simulink model "Maglev_SMC_mfunc"  (R2025a)
settings: Solver=ode23t  StartTime=0.0  StopTime=T_sim  FixedStep=ekf_params.Ts  MaxStep=Ts  RelTol=1e-2  AbsTol=1e-4
PreLoadFcn:
  | % Modellpfad abrufen
  | modelPath = fileparts(which(bdroot));
  | projectRoot = fileparts(modelPath);
  | 
  | % Simulationsumgebung einrichten und Parameter laden
  | run(fullfile(projectRoot, 'setup_sim_params.m'));
  | load(fullfile(projectRoot, 'Controller_Params', 'EKFData.mat'));
  | load(fullfile(projectRoot, 'Controller_Params', 'NonlinearControllerData.mat'));
undefined symbols (not defined in the file): ekf_params, Ext_Fina_Val, Ext_Init_Val, grav, I_max, I_min, Km, mass, Plant, smc, T_stp
libraries: fl_lib x11, nesl_utility x4
settings Model: Creator=Polarstern  LastModifiedBy=CelestialAurora
settings DebuggingCC: AlgebraicLoopMsg=none

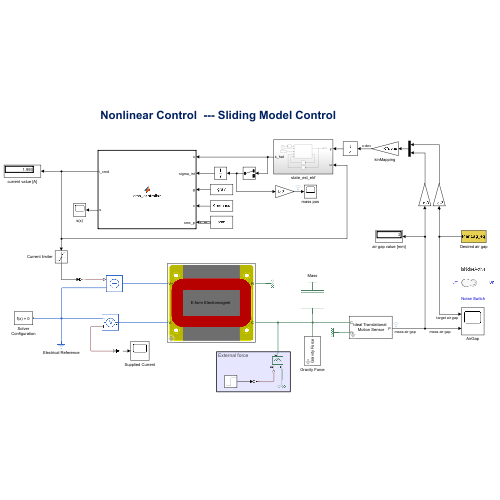
[thumbnail: Simulink's stored preview of the top-level diagram]
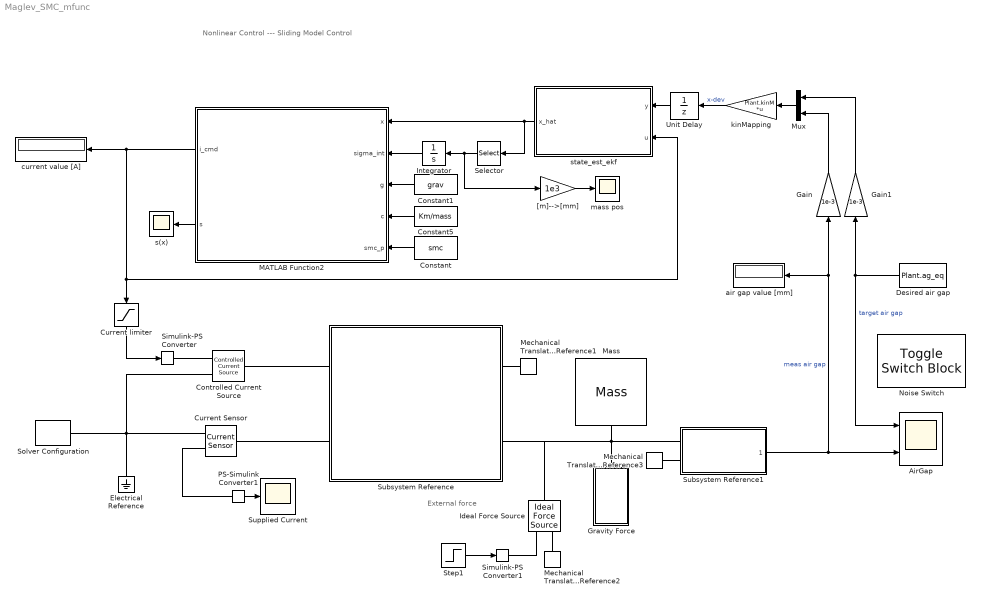
== system Maglev_SMC_mfunc ==
  note: External force
  note: Nonlinear Control --- Sliding Model Control
  AirGap : Scope  NumInputPorts=2
      settings: ActiveDisplayYMinimum=1.7979494790618245  ActiveDisplayYMaximum=2.5780056134375751
  Constant : Constant  Value=smc  OutDataTypeStr=Bus: smc_Bus
  Constant1 : Constant  Value=grav
  Constant5 : Constant  Value=Km/mass
  Controlled Current Source : fl_lib/Electrical/Electrical Sources/Controlled Current Source
  Current Sensor : fl_lib/Electrical/Electrical Sensors/Current Sensor
  Current limiter : Saturate  UpperLimit=I_max  LowerLimit=I_min
  Desired air gap : Constant  Value=Plant.ag_eq
  Electrical Reference : fl_lib/Electrical/Electrical Elements/Electrical Reference
  Gain : Gain  Gain=1e-3
  Gain1 : Gain  Gain=1e-3
  Gravity Force : Subsystem
      mask DialogControl DescGroupVar Prompt: Gravity Force
      mask DialogControl DescTextVar Prompt: Fg = Mass*grav, as constant parameters predefined
      mask DialogControl DescTextVar2 Prompt: Direction: Downward
      mask Display: disp("Gravity Force")
  Ideal Force Source : fl_lib/Mechanical/Mechanical Sources/Ideal Force Source
  Integrator : Integrator
  MATLAB Function2 : MATLAB Function  TreatAsAtomicUnit=on
  Mass : fl_lib/Mechanical/Translational Elements/Mass  mass=mass kg  num_ports=foundation.enum.numPorts2.one  v_specify=on  v_priority=Low  v=0 m/s  v_nominal_specify=off  v_nominal_value=1  v_nominal_unit=m/s  f_specify=off  f_priority=None  f=0 N  f_nominal_specify=off  f_nominal_value=700  f_nominal_unit=N
  Mechanical Translational Reference1 : fl_lib/Mechanical/Translational Elements/Mechanical Translational Reference
  Mechanical Translational Reference2 : fl_lib/Mechanical/Translational Elements/Mechanical Translational Reference
  Mechanical Translational Reference3 : fl_lib/Mechanical/Translational Elements/Mechanical Translational Reference
  Mux : Mux  Inputs=2
  Noise Switch : ToggleSwitchBlock
  PS-Simulink Converter1 : nesl_utility/PS-Simulink Converter  PhysicalDomain=network_engine_domain  SubClassName=ps_output  LeftPortType=input  RightPortType=output  PseudoPeriodic=off  Frequencies=[]  VectorFormat=inherit  Unit=inherit  AffineConversion=off
  Selector : Selector  InputPortWidth=2  IndexOptions=Index vector (dialog)  Indices=[1]  OutputSizes=1
  Simulink-PS Converter : nesl_utility/Simulink-PS Converter  PhysicalDomain=network_engine_domain  SubClassName=ps_input  LeftPortType=input  RightPortType=output  PseudoPeriodic=off  Frequencies=[]  NoiseDistribution=none  NoiseParameters=[]  Unit=1  AffineConversion=off  FilteringAndDerivatives=zero  SimscapeFilterOrder=1  InputFilterTimeConstant=0.001  UdotUserProvided=0
  Simulink-PS Converter1 : nesl_utility/Simulink-PS Converter  PhysicalDomain=network_engine_domain  SubClassName=ps_input  LeftPortType=input  RightPortType=output  PseudoPeriodic=off  Frequencies=[]  NoiseDistribution=none  NoiseParameters=[]  Unit=1  AffineConversion=off  FilteringAndDerivatives=provide  SimscapeFilterOrder=1  InputFilterTimeConstant=0.001  UdotUserProvided=0
  Solver Configuration : nesl_utility/Solver Configuration  PhysicalDomain=network_engine_domain  SubClassName=solver  LeftPortType=input  RightPortType=generic  Tones=[]  Harmonics=[]  SimulateNoise=off  Profile=off  UseLocalSampling=off  EnableSwitchedLinearOptims=on  FrequencyDomain=off  UseCCode=off  RelTol=0.001  AbsTol=1e-06  MinStep=1e-09  ToWorkspace=off  RevertToSquareIcSolve=off  NumHomotopyIterations=100  PhasorMode=off  PhasorModeNumHarmonics=1  ConsistencySolver=NEWTON_XTOL_AFTER_FTOL  IndexReductionMethod=DerivativeReplacement  DoDC=off  ResidualTolerance=1e-09  ConsistencyTolSource=GLOBAL  ConsistencyAbsTol=0.001  ConsistencyRelTol=0.001  ConsistencyTolFactor=0.001  UseLocalSolver=on  LocalSolverChoice=NE_BACKWARD_EULER_ADVANCER  ResolveIndetEquations=on  FunctionEvalNumThread=1  LocalSolverSampleTime=ekf_params.Ts  DoFixedCost=off  MaxNonlinIter=3  MaxModeIter=2  ComputeImpulses=off  ImpulseIterations=2  LinearAlgebra=auto  LinearAlgebraNumThread=0  EquationFormulation=NE_TIME_EF  DelaysMemoryBudget=1024  AutomaticFiltering=on  FilteringTimeConstant=0.001  PartitionStorageMethod=AS_NEEDED  PartitionMemoryBudget=1024  PartitionMethod=ROBUST  MultibodyUseLocalSolver=off  MultibodyLocalSolverChoice=ODE1  MultibodyLocalSolverSampleTime=0.001
  Step1 : Step  Time=T_stp  Before=Ext_Init_Val  After=Ext_Fina_Val  SampleTime=0
  Subsystem Reference : Subsystem  ReferencedSubsystem=IntegratedElectromagnet  l_airgap=airgap_init
  Subsystem Reference1 : Subsystem  ReferencedSubsystem=IdealTrans_MotionSensor  ns_sw=isNoiseActive  ns_pw=NoisePower  ts=Ts  init_pos=airgap_init
  Supplied Current : Scope
      settings: ActiveDisplayYMinimum=-1.1586536453243705  ActiveDisplayYMaximum=10.427882807919337  DataLoggingVariableName=ScopeData3
  Unit Delay : UnitDelay  SampleTime=-1  HasFrameUpgradeWarning=on
  "[m]-->[mm]" : Gain  Gain=1e3
  air gap value [mm] : Display
      settings: Decimation=4
  current value [A] : Display
  kinMapping : Gain  Gain=Plant.kinM  Multiplication=Matrix(K*u) (u vector)
  mass pos : Scope
      settings: ActiveDisplayYMinimum=-0.61398776345659289  ActiveDisplayYMaximum=0.23315599711569898  DataLoggingVariableName=ScopeData4
  s(x) : Scope
      settings: ActiveDisplayYMinimum=-0.38506870213892974  ActiveDisplayYMaximum=0.11483600786407766  DataLoggingVariableName=ScopeData2
  state_est_ekf : Subsystem
  wires:
  Current limiter/1 -> Simulink-PS Converter/1
  PS-Simulink Converter1/1 -> Supplied Current/1
  Step1/1 -> Simulink-PS Converter1/1
  Constant/1 -> MATLAB Function2/5(smc_p)
  Constant1/1 -> MATLAB Function2/3(g)
  state_est_ekf/1(x_hat) -> Selector/1, MATLAB Function2/1(x)
  MATLAB Function2/1(i_cmd) -> current value [A]/1, Current limiter/1, state_est_ekf/2(u)
  MATLAB Function2/2(s) -> s(x)/1
  kinMapping/1 -> Unit Delay/1  "x-dev"
  Selector/1 -> Integrator/1, "[m]-->[mm]"/1
  "[m]-->[mm]"/1 -> mass pos/1
  Gain1/1 -> Mux/1
  Subsystem Reference1/1 -> AirGap/2, air gap value [mm]/1, Gain/1  "meas air gap"
  Mux/1 -> kinMapping/1
  Gain/1 -> Mux/2
  Desired air gap/1 -> AirGap/1, Gain1/1  "target air gap"
  Unit Delay/1 -> state_est_ekf/1(y)
  Constant5/1 -> MATLAB Function2/4(c)
  Integrator/1 -> MATLAB Function2/2(sigma_int)
  connections:
  Gravity Force/RConn1 -- Subsystem Reference1/LConn1 -- Ideal Force Source/LConn1 -- Subsystem Reference/RConn2 -- Mass/LConn1
  Current Sensor/RConn2 -- Electrical Reference/LConn1 -- Solver Configuration/RConn1 -- Controlled Current Source/RConn2
  Subsystem Reference/LConn1 -- Controlled Current Source/LConn1
  Subsystem Reference/LConn2 -- Current Sensor/LConn1
  Simulink-PS Converter/RConn1 -- Controlled Current Source/RConn1
  PS-Simulink Converter1/LConn1 -- Current Sensor/RConn1
  Subsystem Reference/RConn1 -- Mechanical Translational Reference1/LConn1
  Simulink-PS Converter1/RConn1 -- Ideal Force Source/RConn1
  Mechanical Translational Reference2/LConn1 -- Ideal Force Source/RConn2
  Mechanical Translational Reference3/LConn1 -- Subsystem Reference1/LConn2

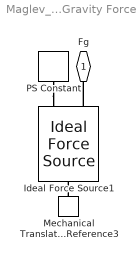
== system Maglev_SMC_mfunc/Gravity Force ==
  Ideal Force Source1 : fl_lib/Mechanical/Mechanical Sources/Ideal Force Source
  Mechanical Translational Reference3 : fl_lib/Mechanical/Translational Elements/Mechanical Translational Reference
  PS Constant : fl_lib/Physical Signals/Sources/PS Constant  constant=mass*grav N
  Fg : PMIOPort  Side=Right
  connections:
  Mechanical Translational Reference3/LConn1 -- Ideal Force Source1/LConn1
  PS Constant/RConn1 -- Ideal Force Source1/RConn1
  Ideal Force Source1/RConn2 -- Fg/RConn1

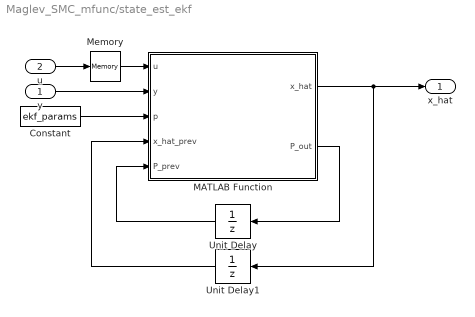
== system Maglev_SMC_mfunc/state_est_ekf ==
  y : Inport
  u : Inport  Port=2
  Constant : Constant  Value=ekf_params  OutDataTypeStr=Bus: ekf_Bus
  MATLAB Function : MATLAB Function  TreatAsAtomicUnit=on
  Memory : Memory  InitialCondition=ekf_params.u0
  Unit Delay : UnitDelay  InitialCondition=ekf_params.P0  SampleTime=-1  HasFrameUpgradeWarning=on
  Unit Delay1 : UnitDelay  InitialCondition=ekf_params.x0  SampleTime=-1  HasFrameUpgradeWarning=on
  x_hat : Outport
  wires:
  MATLAB Function/2(P_out) -> Unit Delay/1
  MATLAB Function/1(x_hat) -> x_hat/1, Unit Delay1/1
  Constant/1 -> MATLAB Function/3(p)
  Unit Delay1/1 -> MATLAB Function/4(x_hat_prev)
  Unit Delay/1 -> MATLAB Function/5(P_prev)
  y/1 -> MATLAB Function/2(y)
  u/1 -> Memory/1
  Memory/1 -> MATLAB Function/1(u)

== matlab function Maglev_SMC_mfunc/state_est_ekf/MATLAB Function ==
  data: u input; y input; p input; x_hat output; x_hat_prev input; P_prev input; P_out output
function [x_hat, P_out] = ekf_maglev(u, y, p, x_hat_prev, P_prev)
    % EKF for single-magnet levitation system
    %
    % Inputs:
    %   y           - measured position deviation x1 (scalar, with noise)
    %   u           - applied current i_s (scalar, control input)
    %   x_hat_prev  - state estimate from previous step [x1_hat; x2_hat]
    %   P_prev      - covariance from previous step (2x2)
    %   Km, m, g    - plant parameters
    %   x0          - nominal air gap (2e-3 m)
    %   Ts          - sample period
    %   Q           - process noise covariance (2x2, design parameter)
    %   R           - measurement noise covariance (scalar, sensor spec)
    %
    % Outputs:
    %   x_hat       - updated state estimate [x1_hat; x2_hat]
    %   P_out       - updated covariance (2x2)
    
    Ts = p.Ts;  Q = p.Q;  R = p.R;  H = p.H;
    Km = p.Km;  m = p.m;  g = p.g;  x0 = p.x_gap;

    %% --- 1. Predict step ---
    % Evaluate nonlinear dynamics at previous estimate
    x1 = x_hat_prev(1);
    x2 = x_hat_prev(2);
    
    % Guard against numerical issues if estimate drifts toward magnet
    gap = max(x0 - x1, 1e-9);
    
    % Predicted state (Euler integration of nonlinear dynamics)
    x_pred = [ x1 + Ts * x2;
               x2 + Ts * ( (Km/m) * u^2 / gap^2 - g ) ];
    
    % Jacobian F evaluated at previous estimate
    F = [ 1,                                    Ts;
          Ts * 2 * Km * u^2 / (m * gap^3),       1  ];
    
    % Predicted covariance
    P_pred = F * P_prev * F' + Q;
    
    %% --- 2. Update step ---
    % H = [1, 0];                  % measure position only
    
    % Innovation
    y_pred = H * x_pred;
    innov  = y - y_pred;
    
    % Innovation covariance
    S = H * P_pred * H' + R;
    
    % Kalman gain
    K = (P_pred * H') / S;
    
    % Corrected state and covariance
    x_hat = x_pred + K * innov;
    P_out = (eye(2) - K * H) * P_pred;
    
    % Symmetrize to fight numerical drift
    P_out = 0.5 * (P_out + P_out');
end

== matlab function Maglev_SMC_mfunc/MATLAB Function2 ==
  data: x input; sigma_int input; g input; c input; i_cmd output; smc_p input; s output
function [i_cmd, s] = smc_controller(x, sigma_int, g, c, smc_p)
%% SMC with integral sliding surface
%
% Inputs:
%   x         - [x1; x2] state vector (2×1): position deviation [m], velocity [m/s]
%   sigma_int - integral of x1 (scalar), fed from external Simulink integrator
%   c         - Km/m  [N·m²/A²/kg]
%   grav      - gravity 9.81  [m/s²]
%   smc_p     - parameter struct:
%                 .x0      equilibrium air gap [m]
%                 .lambda  sliding surface coefficient [rad/s]
%                 .eta     saturation reaching gain
%                 .K       exponential reaching gain
%                 .phi     boundary layer width
%                 .ki      integral gain (set 0 to disable)
%
% Outputs:
%   i_cmd - commanded current [A]
%   s     - sliding surface value (connect to scope for tuning)

    x1 = x(1);    % position deviation [m]
    x2 = x(2);    % velocity [m/s]

    %% Integral sliding surface
    %   Original:  s = lambda*x1 + x2
    %   Extended:  s = lambda*x1 + x2 + ki*sigma_int
    s = smc_p.lambda * x1 + x2 + smc_p.ki * sigma_int;

    %% System terms
    x_gap = max(smc_p.x0 - x1, 1e-6);

    % C^T * f(x) — gains ki*x1 term because:
    %   d/dt(s) = lambda*x2 + x2_dot + ki*x1
    %           = lambda*x2 + [f(x) + g(x)*u] + ki*x1
    % so the feedforward must cancel lambda*x2 - grav + ki*x1
    CTf = smc_p.lambda * x2 - g + smc_p.ki * x1;

    CTg = c / x_gap^2;

    %% Reaching law (unchanged)
    sat_s = max(-1, min(1, s / smc_p.phi));
    h_s   = -smc_p.eta * sat_s - smc_p.K * s;

    %% Control law
    u     = (-CTf + h_s) / CTg;
    u     = max(u, 0);
    i_cmd = sqrt(u);
end
